simulink model "SC_CL_model"  (R2025b)
settings: Solver=VariableStepAuto  StartTime=0.0  StopTime=10.0  RelTol=1e-3
undefined symbols (not defined in the file or in its folder): APE, Kp_x, Kp_y, Kp_z, Kv_x, Kv_y, Kv_z, PSD_GYRO, PSD_SST, Tpert, w_x, w_y, w_z
libraries: cstblocks x4, RCTblocks x1
settings Model: Creator=d.alazard  LastModifiedBy=andre
settings SolverCC: AlgebraicLoopSolver=TrustRegion
settings DataIOCC: ReturnWorkspaceOutputs=off
settings DebuggingCC: AlgebraicLoopMsg=none  UnconnectedInputMsg=warning  UnconnectedOutputMsg=warning  UnconnectedLineMsg=warning  ArithmeticOperatorsInVariantConditions=warning
settings ModelReferenceCC: EnableRefExpFcnMdlSchedulingChecks=on
settings SFSimCC: CustomCodeUndefinedFunction=UseInterfaceOnly
settings RTWCC: GPUComputeCapability=3.5  DLArmComputeVersion=19.05

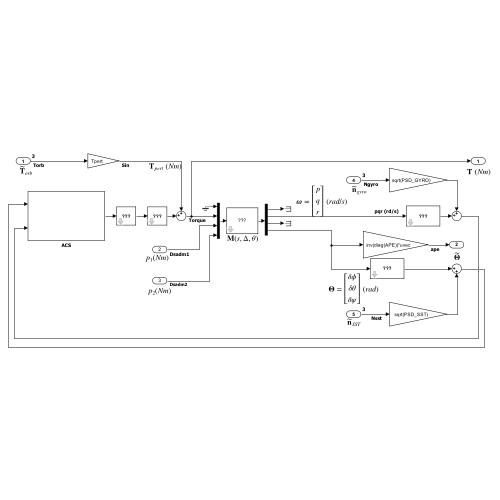
[thumbnail: Simulink's stored preview of the top-level diagram]
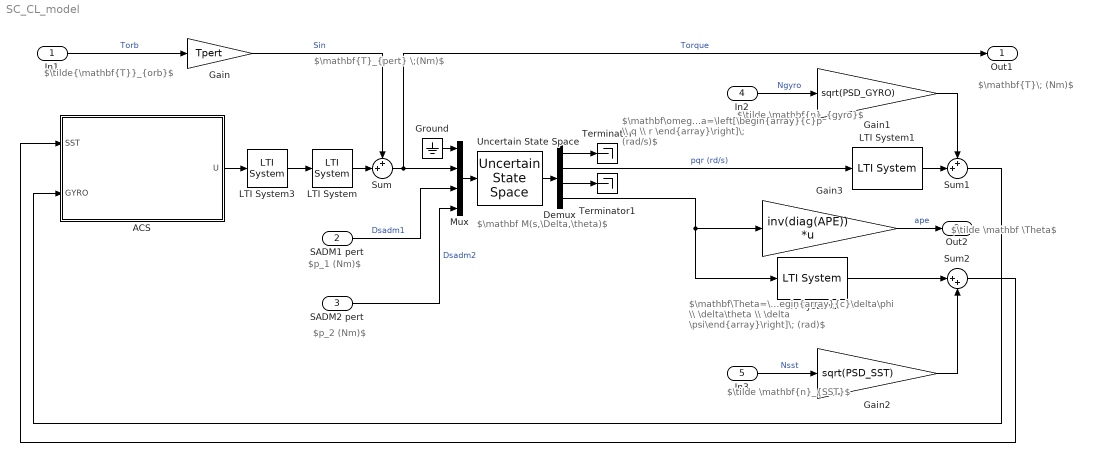
== system SC_CL_model ==
  note: $p_1 (Nm)$
  note: $\mathbf{T}_{pert} \;(Nm)$
  note: $\mathbf M(s,\Delta,\theta)$
  note: $\tilde{\mathbf{T}}_{orb}$
  note: $\mathbf{T}\; (Nm)$
  note: $\mathbf\Theta=\left[\begin{array}{c}\delta\phi \\ \delta\theta \\ \delta \psi\end{array}\right]\; (rad)$
  note: $\tilde \mathbf \Theta$
  note: $\tilde \mathbf{n}_{gyro}$
  note: $\tilde \mathbf{n}_{SST}$
  note: $p_2 (Nm)$
  note: $\mathbf\omega=\left[\begin{array}{c}p \\ q \\ r \end{array}\right]\; (rad/s)$
  In1 : Inport  PortDimensions=3
  SADM1 pert : Inport  Port=2  PortDimensions=1
  SADM2 pert : Inport  Port=3  PortDimensions=1
  In2 : Inport  Port=4  PortDimensions=3
  In3 : Inport  Port=5  PortDimensions=3
  ACS : Subsystem
  Demux : Demux  Outputs=[9 3 3 3]
  Gain : Gain  Gain=Tpert
  Gain1 : Gain  Gain=sqrt(PSD_GYRO)
  Gain2 : Gain  Gain=sqrt(PSD_SST)
  Gain3 : Gain  Gain=inv(diag(APE))  Multiplication=Matrix(K*u) (u vector)
  Ground : Ground
  LTI System : cstblocks/LTI System  sys=RW  IC=[]  PadeOrder=0
  LTI System1 : cstblocks/LTI System  sys=GYRO  IC=[]  PadeOrder=0
  LTI System2 : cstblocks/LTI System  sys=SST  IC=[]  PadeOrder=0
  LTI System3 : cstblocks/LTI System  sys=DELAY  IC=[]  PadeOrder=0
  Mux : Mux  Inputs=[3 3 1 1]
  Sum : Sum  Inputs=++|
  Sum1 : Sum  Inputs=++|
  Sum2 : Sum  Inputs=|++
  Terminator : Terminator
  Terminator1 : Terminator
  Uncertain State Space : RCTblocks/Uncertain State Space  Tag=USS  SCDEnableBlockLinearizationSpecification=on  USystem=Gu  UValue=[]  X0=[]  uX0=[]
  Out1 : Outport  VectorParamsAs1DForOutWhenUnconnected=off
  Out2 : Outport  Port=2  VectorParamsAs1DForOutWhenUnconnected=off
  wires:
  LTI System/1 -> Sum/2
  Sum/1 -> Mux/2, Out1/1  "Torque"
  In1/1 -> Gain/1  "Torb"
  Demux/2 -> LTI System1/1  "pqr (rd/s)"
  LTI System1/1 -> Sum1/2
  In2/1 -> Gain1/1  "Ngyro"
  Demux/4 -> LTI System2/1, Gain3/1
  Sum2/1 -> ACS/1(SST)
  Sum1/1 -> ACS/2(GYRO)
  ACS/1(U) -> LTI System3/1
  LTI System3/1 -> LTI System/1
  Gain/1 -> Sum/1  "Sin"
  Gain1/1 -> Sum1/1
  In3/1 -> Gain2/1  "Nsst"
  Gain2/1 -> Sum2/2
  LTI System2/1 -> Sum2/1
  Gain3/1 -> Out2/1  "ape"
  Uncertain State Space/1 -> Demux/1
  Demux/1 -> Terminator/1
  SADM2 pert/1 -> Mux/4  "Dsadm2"
  SADM1 pert/1 -> Mux/3  "Dsadm1"
  Ground/1 -> Mux/1
  Mux/1 -> Uncertain State Space/1
  Demux/3 -> Terminator1/1

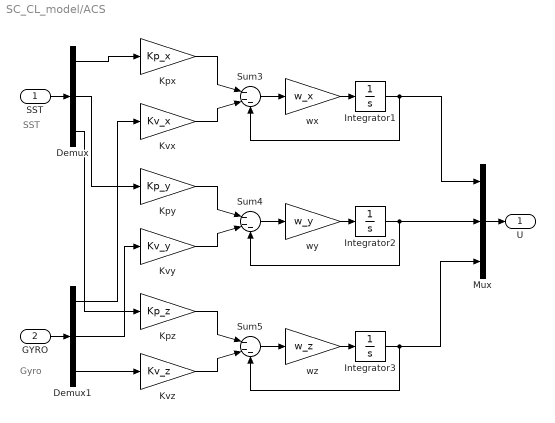
== system SC_CL_model/ACS ==
  note: Gyro
  note: SST
  SST : Inport
  GYRO : Inport  Port=2
  Demux : Demux  Outputs=3
  Demux1 : Demux  Outputs=3
  Integrator1 : Integrator
  Integrator2 : Integrator
  Integrator3 : Integrator
  Kpx : Gain  Gain=Kp_x
  Kpy : Gain  Gain=Kp_y
  "Kpz " : Gain  Gain=Kp_z
  Kvx : Gain  Gain=Kv_x
  Kvy : Gain  Gain=Kv_y
  Kvz : Gain  Gain=Kv_z
  Mux : Mux  Inputs=3
  Sum3 : Sum  Inputs=|---
  Sum4 : Sum  Inputs=|---
  Sum5 : Sum  Inputs=|---
  wx : Gain  Gain=w_x
  wy : Gain  Gain=w_y
  wz : Gain  Gain=w_z
  U : Outport  VectorParamsAs1DForOutWhenUnconnected=off
  wires:
  Kvx/1 -> Sum3/2
  Integrator1/1 -> Sum3/3, Mux/1
  "Kpz "/1 -> Sum5/1
  Integrator3/1 -> Mux/3, Sum5/3
  Mux/1 -> U/1
  Demux1/3 -> Kvz/1
  Kvy/1 -> Sum4/2
  Sum3/1 -> wx/1
  SST/1 -> Demux/1
  Integrator2/1 -> Mux/2, Sum4/3
  Demux/1 -> Kpx/1
  Demux1/1 -> Kvx/1
  Sum5/1 -> wz/1
  Demux/3 -> "Kpz "/1
  GYRO/1 -> Demux1/1
  wy/1 -> Integrator2/1
  Kpy/1 -> Sum4/1
  Demux1/2 -> Kvy/1
  wx/1 -> Integrator1/1
  Demux/2 -> Kpy/1
  Kvz/1 -> Sum5/2
  Sum4/1 -> wy/1
  wz/1 -> Integrator3/1
  Kpx/1 -> Sum3/1
